simulink model "gyro_fusion"  (R2014a)
settings: Solver=VariableStepDiscrete  StartTime=0.0  StopTime=t_sim  MaxStep=0.001  RelTol=1e-3
undefined symbols (not defined in the file): acc_data, diff, gravity_I, gyro_data, magnetometer_data, R_acc, R_gyro, R_magnetometer, ref_B_I
libraries: lib_gyro_fusion x14, vrlib x1
settings Model: Creator=kirill  LastModifiedBy=kirill

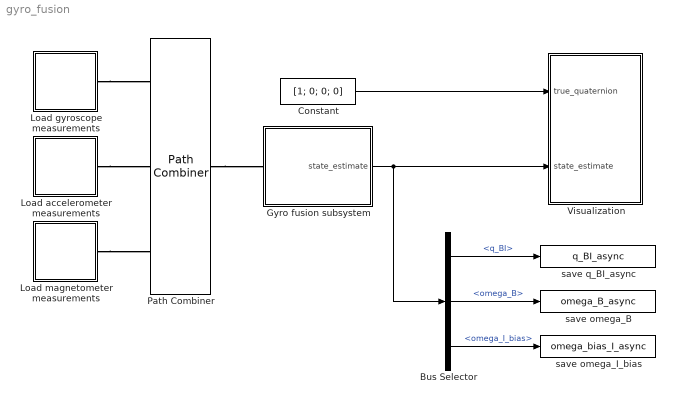
== system gyro_fusion ==
  Bus Selector : BusSelector  OutputSignals=q_BI,omega_B,omega_I_bias
  Constant : Constant  Value=[1; 0; 0; 0]
  Gyro fusion subsystem : Subsystem
  Load accelerometer measurements : Subsystem  mask{measurement_type=2, observed_data=acc_data, R_measurement=R_acc, ref_direction_I=gravity_I}
      mask prompts: measurement_type "Measuerment type (integer identifyer)"; observed_data "Observation data (see from workspace documentation)"; R_measurement "Measurement covariance matrix"; ref_direction_I "Reference direction"
  Load gyroscope measurements : Subsystem  mask{measurement_type=1, observed_data=gyro_data, R_measurement=R_gyro}
      mask prompts: measurement_type "Measuerment type (integer identifyer)"; observed_data "Observation data (see from workspace documentation)"; R_measurement "Measurement covariance matrix"
  Load magnetometer measurements : Subsystem  mask{measurement_type=2, observed_data=magnetometer_data, R_measurement=R_magnetometer, ref_direction_I=ref_B_I}
      mask prompts: measurement_type "Measuerment type (integer identifyer)"; observed_data "Observation data (see from workspace documentation)"; R_measurement "Measurement covariance matrix"; ref_direction_I "Reference direction"
  Path Combiner : PathCombiner
  Visualization : Subsystem
  save omega_B : ToWorkspace  VariableName=omega_B_async  SaveFormat=Timeseries  SampleTime=-1
  save omega_I_bias : ToWorkspace  VariableName=omega_bias_I_async  SaveFormat=Timeseries  SampleTime=-1
  save q_BI_async : ToWorkspace  VariableName=q_BI_async  SaveFormat=Timeseries  SampleTime=-1
  wires:
  Gyro fusion subsystem/1(state_estimate) -> Bus Selector/1, Visualization/2(state_estimate)
  Constant/1 -> Visualization/1(true_quaternion)
  Bus Selector/1 -> save q_BI_async/1  "<q_BI>"
  Bus Selector/3 -> save omega_I_bias/1  "<omega_I_bias>"
  Bus Selector/2 -> save omega_B/1  "<omega_B>"
  connections:
  Load gyroscope measurements/RConn1 -- Path Combiner/LConn1
  Load accelerometer measurements/RConn1 -- Path Combiner/LConn2
  Path Combiner/RConn1 -- Gyro fusion subsystem/LConn1
  Load magnetometer measurements/RConn1 -- Path Combiner/LConn3

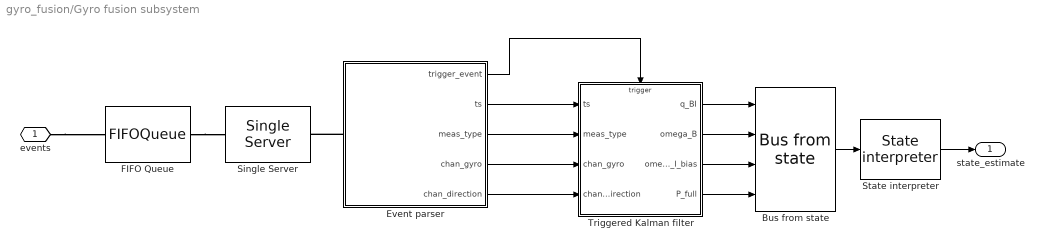
== system gyro_fusion/Gyro fusion subsystem ==
  Bus from state : lib_gyro_fusion/Bus from state
  Event parser : Subsystem
  FIFO Queue : FIFOQueue  Capacity=500
  Single Server : SingleServer  ServiceTime=0.001
  State interpreter : lib_gyro_fusion/State interpreter
  Triggered Kalman filter : Subsystem  TreatAsAtomicUnit=on
  events : PMIOPort  Port=1  Side=Left
  state_estimate : Outport
  wires:
  Triggered Kalman filter/4(P_full) -> Bus from state/4
  Triggered Kalman filter/3(omega_I_bias) -> Bus from state/3
  Event parser/4(chan_gyro) -> Triggered Kalman filter/3(chan_gyro)
  Triggered Kalman filter/2(omega_B) -> Bus from state/2
  Event parser/5(chan_direction) -> Triggered Kalman filter/4(chan_direction)
  Triggered Kalman filter/1(q_BI) -> Bus from state/1
  Bus from state/1 -> State interpreter/1
  State interpreter/1 -> state_estimate/1
  Event parser/1(trigger_event) -> Triggered Kalman filter/Trigger
  Event parser/2(ts) -> Triggered Kalman filter/1(ts)
  Event parser/3(meas_type) -> Triggered Kalman filter/2(meas_type)
  connections:
  events/RConn1 -- FIFO Queue/LConn1
  FIFO Queue/RConn1 -- Single Server/LConn1
  Event parser/LConn1 -- Single Server/RConn1

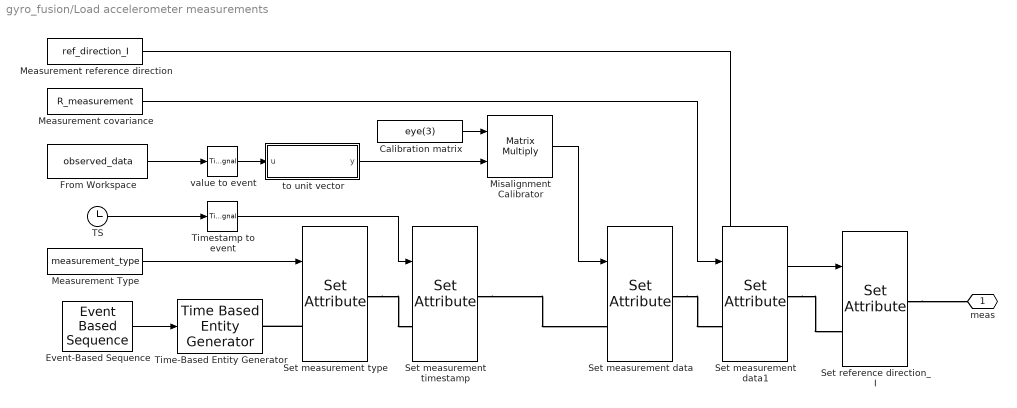
== system gyro_fusion/Load accelerometer measurements ==
  Calibration matrix : Constant  Value=eye(3)
  Event-Based Sequence : EventBasedSequence  VectorOutputValues=diff(observed_data.time)  FormOutputOpt=Setting to infinity
  From Workspace : FromWorkspace  VariableName=observed_data  SampleTime=0
  Measurement Type : Constant  Value=measurement_type
  Measurement covariance : Constant  Value=R_measurement
  Measurement reference direction : Constant  Value=ref_direction_I
  Misalignment Calibrator : Product  Multiplication=Matrix(*)
  Set measurement data : SetAttribute  AttributeName=value  AttributeFrom=Signal port  EvaluatedAttributeValue={ []}
  Set measurement data1 : SetAttribute  AttributeName=R  AttributeFrom=Signal port  EvaluatedAttributeValue={ []}
  Set measurement timestamp : SetAttribute  AttributeName=ts  AttributeFrom=Signal port  EvaluatedAttributeValue={ []}
  Set measurement type : SetAttribute  AttributeName=meas_type  AttributeFrom=Signal port  EvaluatedAttributeValue={ []}
  Set reference direction_I : SetAttribute  AttributeName=ref_direction_I  AttributeFrom=Signal port  EvaluatedAttributeValue={ []}
  TS : Clock
  Time-Based Entity Generator : TimeBasedEntityGenerator  GenerateEntitiesUpon=Intergeneration time from port t
  Timestamp to event : TimedToEventSignal
  to unit vector : MATLAB Function  TreatAsAtomicUnit=on
  value to event : TimedToEventSignal
  meas : PMIOPort  Port=1  Side=Right
  wires:
  TS/1 -> Timestamp to event/1
  From Workspace/1 -> value to event/1
  Event-Based Sequence/1 -> Time-Based Entity Generator/1
  Measurement Type/1 -> Set measurement type/1
  Timestamp to event/1 -> Set measurement timestamp/1
  value to event/1 -> to unit vector/1(u)
  Measurement covariance/1 -> Set measurement data1/1
  Measurement reference direction/1 -> Set reference direction_I/1
  to unit vector/1(y) -> Misalignment Calibrator/2
  Calibration matrix/1 -> Misalignment Calibrator/1
  Misalignment Calibrator/1 -> Set measurement data/1
  connections:
  Set measurement type/LConn1 -- Time-Based Entity Generator/RConn1
  Set measurement type/RConn1 -- Set measurement timestamp/LConn1
  Set measurement timestamp/RConn1 -- Set measurement data/LConn1
  Set measurement data/RConn1 -- Set measurement data1/LConn1
  Set measurement data1/RConn1 -- Set reference direction_I/LConn1
  Set reference direction_I/RConn1 -- meas/RConn1

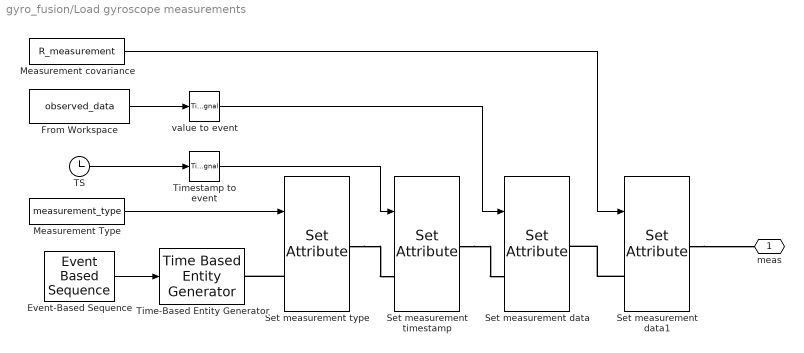
== system gyro_fusion/Load gyroscope measurements ==
  Event-Based Sequence : EventBasedSequence  VectorOutputValues=diff(observed_data.time)  FormOutputOpt=Setting to infinity
  From Workspace : FromWorkspace  VariableName=observed_data  SampleTime=0
  Measurement Type : Constant  Value=measurement_type
  Measurement covariance : Constant  Value=R_measurement
  Set measurement data : SetAttribute  AttributeName=value  AttributeFrom=Signal port  EvaluatedAttributeValue={ []}
  Set measurement data1 : SetAttribute  AttributeName=R  AttributeFrom=Signal port  EvaluatedAttributeValue={ []}
  Set measurement timestamp : SetAttribute  AttributeName=ts  AttributeFrom=Signal port  EvaluatedAttributeValue={ []}
  Set measurement type : SetAttribute  AttributeName=meas_type  AttributeFrom=Signal port  EvaluatedAttributeValue={ []}
  TS : Clock
  Time-Based Entity Generator : TimeBasedEntityGenerator  GenerateEntitiesUpon=Intergeneration time from port t
  Timestamp to event : TimedToEventSignal
  value to event : TimedToEventSignal
  meas : PMIOPort  Port=1  Side=Right
  wires:
  TS/1 -> Timestamp to event/1
  From Workspace/1 -> value to event/1
  Event-Based Sequence/1 -> Time-Based Entity Generator/1
  Measurement Type/1 -> Set measurement type/1
  Timestamp to event/1 -> Set measurement timestamp/1
  Measurement covariance/1 -> Set measurement data1/1
  value to event/1 -> Set measurement data/1
  connections:
  Set measurement type/LConn1 -- Time-Based Entity Generator/RConn1
  Set measurement data1/RConn1 -- meas/RConn1
  Set measurement type/RConn1 -- Set measurement timestamp/LConn1
  Set measurement timestamp/RConn1 -- Set measurement data/LConn1
  Set measurement data1/LConn1 -- Set measurement data/RConn1

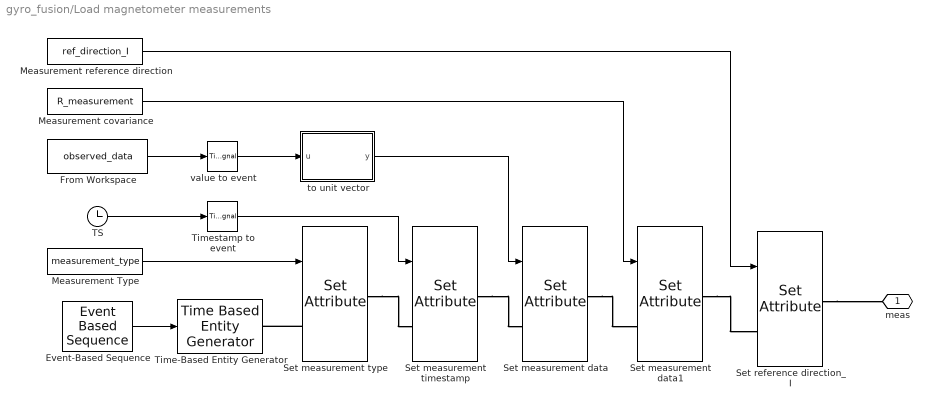
== system gyro_fusion/Load magnetometer measurements ==
  Event-Based Sequence : EventBasedSequence  VectorOutputValues=diff(observed_data.time)  FormOutputOpt=Setting to infinity
  From Workspace : FromWorkspace  VariableName=observed_data  SampleTime=0
  Measurement Type : Constant  Value=measurement_type
  Measurement covariance : Constant  Value=R_measurement
  Measurement reference direction : Constant  Value=ref_direction_I
  Set measurement data : SetAttribute  AttributeName=value  AttributeFrom=Signal port  EvaluatedAttributeValue={ []}
  Set measurement data1 : SetAttribute  AttributeName=R  AttributeFrom=Signal port  EvaluatedAttributeValue={ []}
  Set measurement timestamp : SetAttribute  AttributeName=ts  AttributeFrom=Signal port  EvaluatedAttributeValue={ []}
  Set measurement type : SetAttribute  AttributeName=meas_type  AttributeFrom=Signal port  EvaluatedAttributeValue={ []}
  Set reference direction_I : SetAttribute  AttributeName=ref_direction_I  AttributeFrom=Signal port  EvaluatedAttributeValue={ []}
  TS : Clock
  Time-Based Entity Generator : TimeBasedEntityGenerator  GenerateEntitiesUpon=Intergeneration time from port t
  Timestamp to event : TimedToEventSignal
  to unit vector : MATLAB Function  TreatAsAtomicUnit=on
  value to event : TimedToEventSignal
  meas : PMIOPort  Port=1  Side=Right
  wires:
  TS/1 -> Timestamp to event/1
  From Workspace/1 -> value to event/1
  Event-Based Sequence/1 -> Time-Based Entity Generator/1
  Measurement Type/1 -> Set measurement type/1
  Timestamp to event/1 -> Set measurement timestamp/1
  value to event/1 -> to unit vector/1(u)
  Measurement covariance/1 -> Set measurement data1/1
  Measurement reference direction/1 -> Set reference direction_I/1
  to unit vector/1(y) -> Set measurement data/1
  connections:
  Set measurement type/LConn1 -- Time-Based Entity Generator/RConn1
  Set measurement type/RConn1 -- Set measurement timestamp/LConn1
  Set measurement timestamp/RConn1 -- Set measurement data/LConn1
  Set measurement data/RConn1 -- Set measurement data1/LConn1
  Set measurement data1/RConn1 -- Set reference direction_I/LConn1
  Set reference direction_I/RConn1 -- meas/RConn1

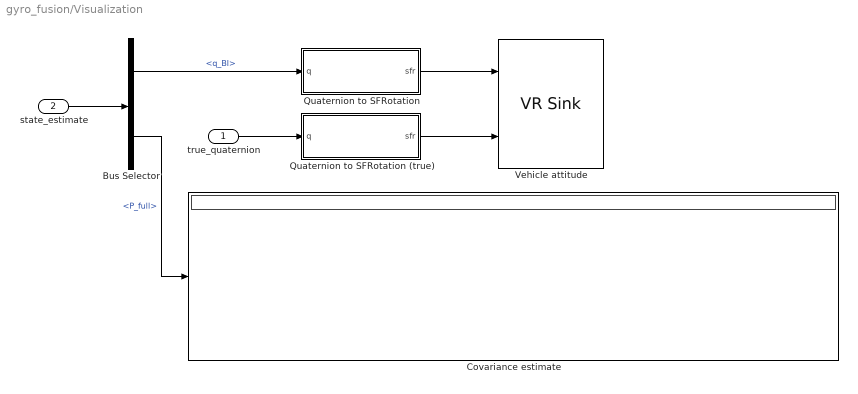
== system gyro_fusion/Visualization ==
  true_quaternion : Inport
  state_estimate : Inport  Port=2
  Bus Selector : BusSelector  OutputSignals=q_BI,P_full
  Covariance estimate : Display
  Quaternion to SFRotation : MATLAB Function  TreatAsAtomicUnit=on
  Quaternion to SFRotation (true) : MATLAB Function  TreatAsAtomicUnit=on
  Vehicle attitude : vrlib/VR Sink  InstantiateOnLoad=on  SampleTime=0.1  ViewEnable=on  RemoteChange=off  RemoteView=off  FieldsWritten=Estimated_car.rotation.4.1.1.double#True_car.rotation.4.1.1.double  WorldFileName=ins.wrl  AutoView=off  VideoDimensions=[]  AllowVariableSize=off
  wires:
  Bus Selector/2 -> Covariance estimate/1  "<P_full>"
  state_estimate/1 -> Bus Selector/1
  Bus Selector/1 -> Quaternion to SFRotation/1(q)  "<q_BI>"
  Quaternion to SFRotation (true)/1(sfr) -> Vehicle attitude/2
  Quaternion to SFRotation/1(sfr) -> Vehicle attitude/1
  true_quaternion/1 -> Quaternion to SFRotation (true)/1(q)

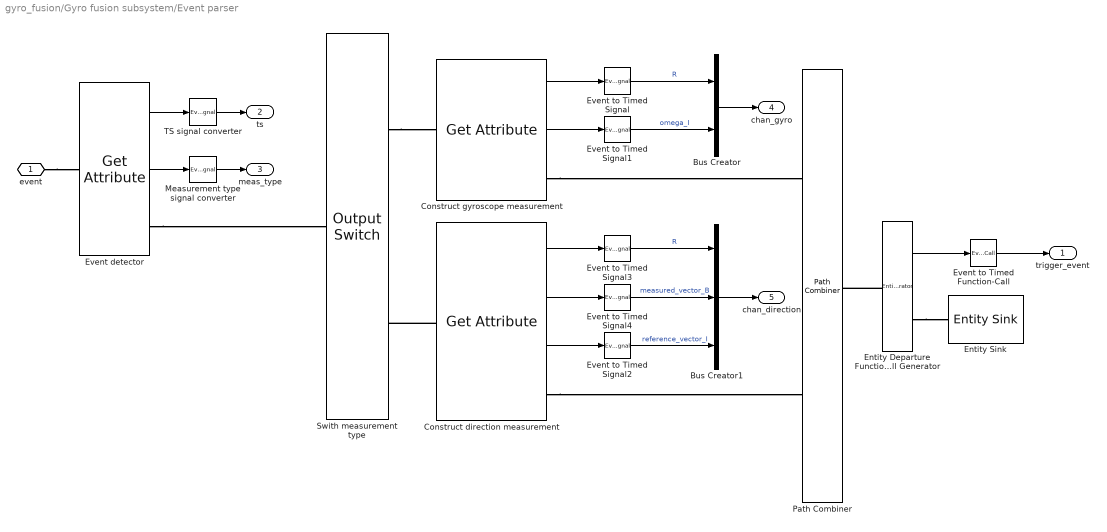
== system gyro_fusion/Gyro fusion subsystem/Event parser ==
  Bus Creator : BusCreator  Inputs=2
  Bus Creator1 : BusCreator  Inputs=3
  Construct direction measurement : GetAttribute  AttributeName=R|value|ref_direction_I  AttributeMissing=Error|Error|Error  AttributeDefaultValue=1|1|1  AttributeTreatAsVector=1|1|1  AttributeSendTiming=After entity departure|After entity departure|After entity departure  EvaluatedDefaultAttributeValue={ [];[];[]}
      settings: OutputPortMap=o1,o2,o3
  Construct gyroscope measurement : GetAttribute  AttributeName=R|value  AttributeMissing=Error|Error  AttributeDefaultValue=1|1  AttributeTreatAsVector=1|1  AttributeSendTiming=After entity departure|After entity departure  EvaluatedDefaultAttributeValue={ [];[]}
      settings: OutputPortMap=o1,o2
  Entity Departure Function-Call Generator : EntityDepartureFunctionCallGenerator
  Entity Sink : EntitySink
  Event detector : GetAttribute  AttributeName=ts|meas_type  AttributeMissing=Error|Error  AttributeDefaultValue=1|1  AttributeTreatAsVector=1|1  AttributeSendTiming=After entity departure|After entity departure  EvaluatedDefaultAttributeValue={ [];[]}
      settings: OutputPortMap=o1,o2
  Event to Timed Signal{,1..4} (5 alike) : EventToTimedSignal
  Event to Timed Function-Call : EventToTimedFunctionCall
  Measurement type signal converter : EventToTimedSignal
  Path Combiner : PathCombiner  NumberInputPorts=2
  Swith measurement type : OutputSwitch  NumberOutputPorts=2  SwitchingCriterion=From attribute  AttributeName=meas_type
  TS signal converter : EventToTimedSignal
  event : PMIOPort  Port=1  Side=Left
  trigger_event : Outport
  ts : Outport  Port=2
  meas_type : Outport  Port=3
  chan_gyro : Outport  Port=4
  chan_direction : Outport  Port=5
  wires:
  Construct gyroscope measurement/2 -> Event to Timed Signal1/1
  Construct gyroscope measurement/1 -> Event to Timed Signal/1
  Construct direction measurement/1 -> Event to Timed Signal3/1
  Bus Creator/1 -> chan_gyro/1
  Bus Creator1/1 -> chan_direction/1
  Construct direction measurement/2 -> Event to Timed Signal4/1
  Event to Timed Signal/1 -> Bus Creator/1  "R"
  Event to Timed Signal1/1 -> Bus Creator/2  "omega_I"
  Event to Timed Signal2/1 -> Bus Creator1/3  "reference_vector_I"
  Event to Timed Signal3/1 -> Bus Creator1/1  "R"
  Event to Timed Signal4/1 -> Bus Creator1/2  "measured_vector_B"
  Construct direction measurement/3 -> Event to Timed Signal2/1
  Entity Departure Function-Call Generator/1 -> Event to Timed Function-Call/1
  Event to Timed Function-Call/1 -> trigger_event/1
  TS signal converter/1 -> ts/1
  Measurement type signal converter/1 -> meas_type/1
  Event detector/1 -> TS signal converter/1
  Event detector/2 -> Measurement type signal converter/1
  connections:
  Construct gyroscope measurement/RConn1 -- Path Combiner/LConn1
  Swith measurement type/RConn1 -- Construct gyroscope measurement/LConn1
  Construct direction measurement/LConn1 -- Swith measurement type/RConn2
  Construct direction measurement/RConn1 -- Path Combiner/LConn2
  Entity Departure Function-Call Generator/RConn1 -- Entity Sink/LConn1
  Entity Departure Function-Call Generator/LConn1 -- Path Combiner/RConn1
  event/RConn1 -- Event detector/LConn1
  Event detector/RConn1 -- Swith measurement type/LConn1

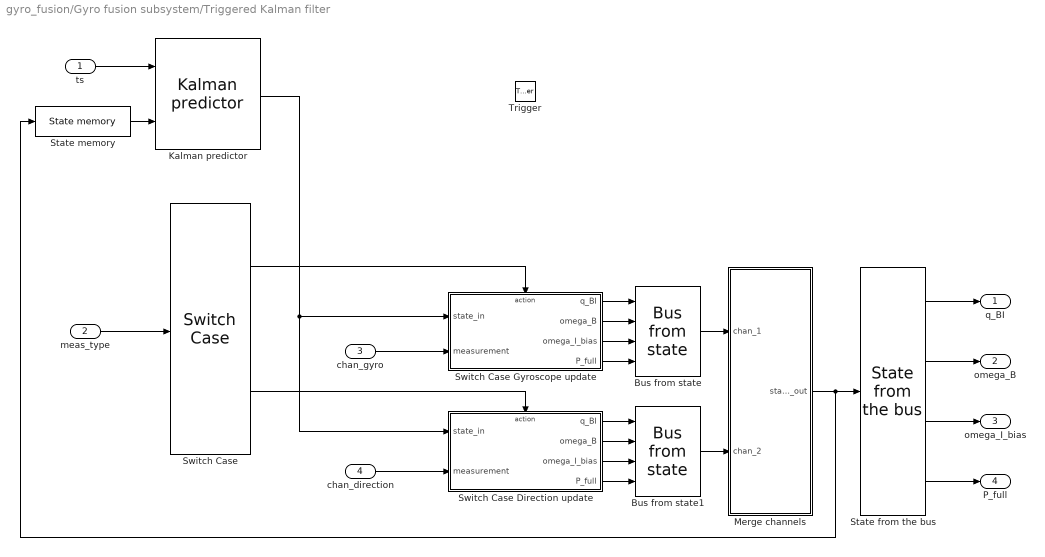
== system gyro_fusion/Gyro fusion subsystem/Triggered Kalman filter ==
  ts : Inport
  meas_type : Inport  Port=2
  chan_gyro : Inport  Port=3
  chan_direction : Inport  Port=4
  Trigger : TriggerPort  TriggerType=function-call
  Bus from state : lib_gyro_fusion/Bus from state
  Bus from state1 : lib_gyro_fusion/Bus from state
  Kalman predictor : lib_gyro_fusion/Kalman predictor  q_noise=q_noise  omega_B_noise=omega_B_noise  omega_I_bias_noise=omega_bias_I_noise
  Merge channels : Subsystem
  State from the bus : lib_gyro_fusion/State from the bus
  State memory : lib_gyro_fusion/State memory  q_BI_init=[1; 0; 0; 0]  omega_B_init=[0; 0; 0]  omega_I_bias_init=[0; 0; 0]  P_full_init=eye(9)
  Switch Case : SwitchCase  CaseConditions={1,2}  ShowDefaultCase=off
  Switch Case Direction update : Subsystem  TreatAsAtomicUnit=on
  Switch Case Gyroscope update : Subsystem  TreatAsAtomicUnit=on
  q_BI : Outport
  omega_B : Outport  Port=2
  omega_I_bias : Outport  Port=3
  P_full : Outport  Port=4
  wires:
  ts/1 -> Kalman predictor/1
  chan_gyro/1 -> Switch Case Gyroscope update/2(measurement)
  meas_type/1 -> Switch Case/1
  Switch Case/1 -> Switch Case Gyroscope update/Action
  Switch Case/2 -> Switch Case Direction update/Action
  chan_direction/1 -> Switch Case Direction update/2(measurement)
  Bus from state1/1 -> Merge channels/2(chan_2)
  Switch Case Gyroscope update/1(q_BI) -> Bus from state/1
  Switch Case Gyroscope update/2(omega_B) -> Bus from state/2
  Switch Case Gyroscope update/3(omega_I_bias) -> Bus from state/3
  Switch Case Gyroscope update/4(P_full) -> Bus from state/4
  Bus from state/1 -> Merge channels/1(chan_1)
  Switch Case Direction update/1(q_BI) -> Bus from state1/1
  Switch Case Direction update/2(omega_B) -> Bus from state1/2
  Switch Case Direction update/3(omega_I_bias) -> Bus from state1/3
  Switch Case Direction update/4(P_full) -> Bus from state1/4
  State memory/1 -> Kalman predictor/2
  State from the bus/1 -> q_BI/1
  State from the bus/2 -> omega_B/1
  State from the bus/3 -> omega_I_bias/1
  State from the bus/4 -> P_full/1
  Merge channels/1(state_out) -> State memory/1, State from the bus/1
  Kalman predictor/1 -> Switch Case Gyroscope update/1(state_in), Switch Case Direction update/1(state_in)

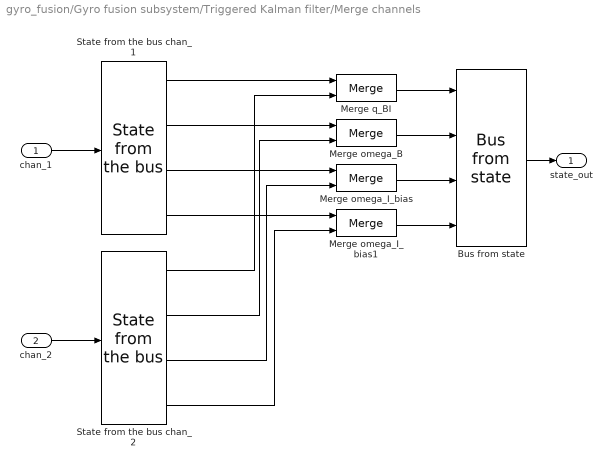
== system gyro_fusion/Gyro fusion subsystem/Triggered Kalman filter/Merge channels ==
  chan_1 : Inport
  chan_2 : Inport  Port=2
  Bus from state : lib_gyro_fusion/Bus from state
  Merge omega_B : Merge
  Merge omega_I_bias : Merge
  Merge omega_I_bias1 : Merge
  Merge q_BI : Merge
  State from the bus chan_1 : lib_gyro_fusion/State from the bus
  State from the bus chan_2 : lib_gyro_fusion/State from the bus
  state_out : Outport
  wires:
  chan_1/1 -> State from the bus chan_1/1
  chan_2/1 -> State from the bus chan_2/1
  State from the bus chan_1/1 -> Merge q_BI/1
  State from the bus chan_1/2 -> Merge omega_B/1
  State from the bus chan_1/3 -> Merge omega_I_bias/1
  State from the bus chan_1/4 -> Merge omega_I_bias1/1
  State from the bus chan_2/1 -> Merge q_BI/2
  State from the bus chan_2/2 -> Merge omega_B/2
  State from the bus chan_2/3 -> Merge omega_I_bias/2
  State from the bus chan_2/4 -> Merge omega_I_bias1/2
  Merge q_BI/1 -> Bus from state/1
  Merge omega_B/1 -> Bus from state/2
  Merge omega_I_bias/1 -> Bus from state/3
  Merge omega_I_bias1/1 -> Bus from state/4
  Bus from state/1 -> state_out/1

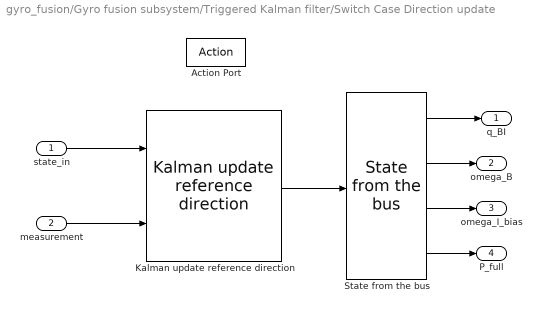
== system gyro_fusion/Gyro fusion subsystem/Triggered Kalman filter/Switch Case Direction update ==
  state_in : Inport
  measurement : Inport  Port=2
  Action Port : ActionPort  ActionType=case
  Kalman update reference direction : lib_gyro_fusion/Kalman update reference direction
  State from the bus : lib_gyro_fusion/State from the bus
  q_BI : Outport
  omega_B : Outport  Port=2
  omega_I_bias : Outport  Port=3
  P_full : Outport  Port=4
  wires:
  state_in/1 -> Kalman update reference direction/1
  measurement/1 -> Kalman update reference direction/2
  State from the bus/4 -> P_full/1
  State from the bus/3 -> omega_I_bias/1
  State from the bus/2 -> omega_B/1
  State from the bus/1 -> q_BI/1
  Kalman update reference direction/1 -> State from the bus/1

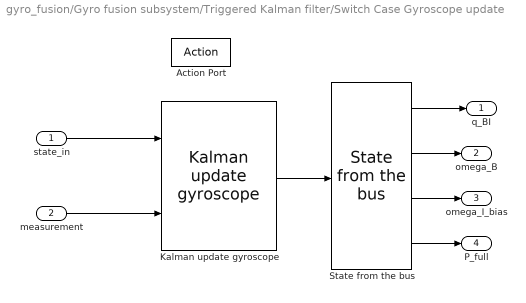
== system gyro_fusion/Gyro fusion subsystem/Triggered Kalman filter/Switch Case Gyroscope update ==
  state_in : Inport
  measurement : Inport  Port=2
  Action Port : ActionPort  ActionType=case
  Kalman update gyroscope : lib_gyro_fusion/Kalman update gyroscope
  State from the bus : lib_gyro_fusion/State from the bus
  q_BI : Outport
  omega_B : Outport  Port=2
  omega_I_bias : Outport  Port=3
  P_full : Outport  Port=4
  wires:
  state_in/1 -> Kalman update gyroscope/1
  measurement/1 -> Kalman update gyroscope/2
  Kalman update gyroscope/1 -> State from the bus/1
  State from the bus/1 -> q_BI/1
  State from the bus/4 -> P_full/1
  State from the bus/3 -> omega_I_bias/1
  State from the bus/2 -> omega_B/1

== matlab function gyro_fusion/Load magnetometer measurements/to unit vector ==
  data: u input; y output
function y = to_unit(u)
%#codegen

y = u / norm(u);

== matlab function gyro_fusion/Load accelerometer measurements/to unit vector ==
  data: u input; y output
function y = to_unit(u)
%#codegen

y = u / norm(u);

== matlab function gyro_fusion/Visualization/Quaternion to SFRotation ==
  data: q input; sfr output
function sfr = quaternion2rotation(q)
%#codegen

sfr = zeros(size(q));
sfr(1:3) = q(2:4);
sfr(4) = 2 * acos(q(1));

== matlab function gyro_fusion/Visualization/Quaternion to SFRotation (true) ==
  data: q input; sfr output
function sfr = quaternion2rotation(q)
%#codegen

sfr = zeros(size(q));
sfr(1:3) = q(2:4);
sfr(4) = 2 * acos(q(1));
